simulink model "twolevel_seriesparallel"  (R2016a)
settings: Solver=VariableStepAuto  StartTime=0.0  StopTime=stop_time  RelTol=1e-3  AbsTol=1e-6
values from neighbouring files (symbols this model uses):
  DCLINK_Cap = 0.65*1.35*capacitorsabiti/sw_frequency    (= 0.000406115702479)    [loadvariation.m]    (also in trials.m = 1.35*capacitorsabiti/sw_frequency; twolevel_seriesparallel_analysis.m)
  Ef = Vln_rms*cos(Load_Angle)    [loadvariation.m]    (also in trials.m; twolevel_seriesparallel_analysis.m)
  intangle1 = 0    [loadvariation.m]    (also in trials.m; twolevel_seriesparallel_analysis.m)
  intangle2 = interleaving_angle    (= 180)    [loadvariation.m]    (also in trials.m = 360; twolevel_seriesparallel_analysis.m)
  intangle3 = 0    [loadvariation.m]    (also in trials.m; twolevel_seriesparallel_analysis.m)
  intangle4 = interleaving_angle    (= 180)    [loadvariation.m]    (also in trials.m = 360; twolevel_seriesparallel_analysis.m)
  Load_Angle = acos(Load_Power_Factor)    [loadvariation.m]    (also in trials.m; twolevel_seriesparallel_analysis.m)
  Ls = n*m*Xs/ref_frequency    [loadvariation.m]    (also in trials.m; twolevel_seriesparallel_analysis.m)
  ma = 0.9    [loadvariation.m]    (also in trials.m; twolevel_seriesparallel_analysis.m)
  ref_frequency = 2*pi*50    (= 314.159265359)    [loadvariation.m]    (also in trials.m; twolevel_seriesparallel_analysis.m)
  Sampling_time = 1/(100*sw_frequency)    (= 1.65289256198e-06)    [loadvariation.m]    (also in twolevel_seriesparallel_analysis.m = 8.26446280992e-06)
  Vin = DC_Voltage_Source + Rin*(Load_Real_Power/DC_Voltage_Source)    (= 554.814814815)    [loadvariation.m]    (also in trials.m; twolevel_seriesparallel_analysis.m)
undefined symbols (not defined in the file or in its folder): intangle5, intangle6, intangle7, intangle8, Lload, Rload
libraries: powerlib x106, powerlib_meascontrol x58, simulink x24
(part 2 of 2)

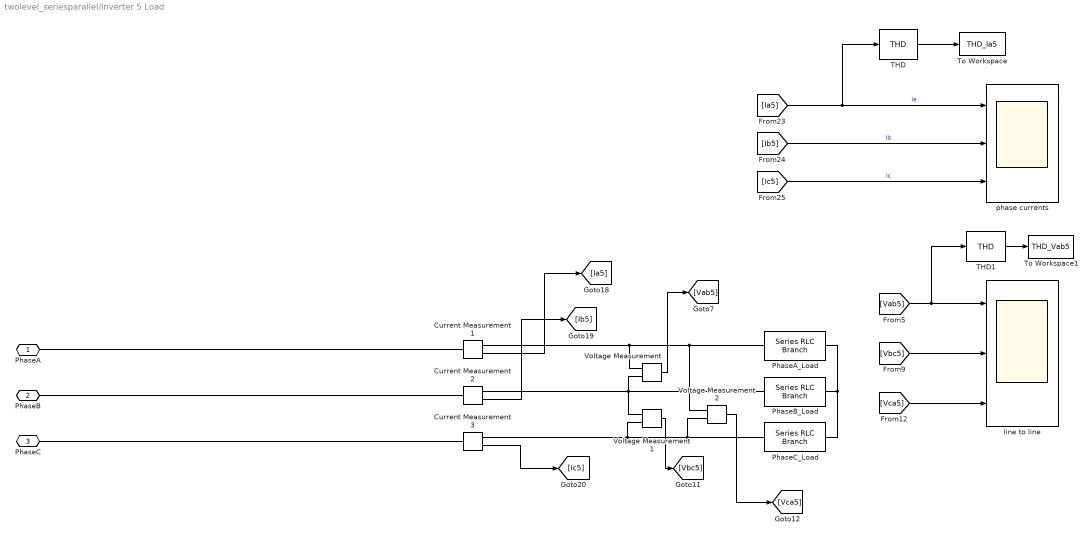
== system twolevel_seriesparallel/Inverter 5 Load ==
  Current Measurement1 : powerlib/Measurements/Current Measurement  PhasorSimulation=off  OutputType=Complex  PSBequivalent=0
  Current Measurement2 : powerlib/Measurements/Current Measurement  PhasorSimulation=off  OutputType=Complex  PSBequivalent=0
  Current Measurement3 : powerlib/Measurements/Current Measurement  PhasorSimulation=off  OutputType=Complex  PSBequivalent=0
  PhaseA_Load : powerlib/Elements/Series RLC Branch  LConnTagsString=__new0  RConnTagsString=__new0  BranchType=RL  Resistance=Rload  Inductance=Lload  SetiL0=off  InitialCurrent=0  Capacitance=1e-6  Setx0=off  InitialVoltage=0  Measurements=None
  PhaseB_Load : powerlib/Elements/Series RLC Branch  LConnTagsString=__new0  RConnTagsString=__new0  BranchType=RL  Resistance=Rload  Inductance=Lload  SetiL0=off  InitialCurrent=0  Capacitance=1e-6  Setx0=off  InitialVoltage=0  Measurements=None
  PhaseC_Load : powerlib/Elements/Series RLC Branch  LConnTagsString=__new0  RConnTagsString=__new0  BranchType=RL  Resistance=Rload  Inductance=Lload  SetiL0=off  InitialCurrent=0  Capacitance=1e-6  Setx0=off  InitialVoltage=0  Measurements=None
  THD : powerlib_meascontrol/Measurements/THD  Freq=Load_Nominal_Freq  Ts=0
  THD1 : powerlib_meascontrol/Measurements/THD  Freq=Load_Nominal_Freq  Ts=0
  To Workspace : ToWorkspace  VariableName=THD_Ia5  SaveFormat=Timeseries  SampleTime=-1
  To Workspace1 : ToWorkspace  VariableName=THD_Vab5  SaveFormat=Timeseries  SampleTime=-1
  Voltage Measurement : powerlib/Measurements/Voltage Measurement  PhasorSimulation=off  OutputType=Complex  PSBequivalent=0
  Voltage Measurement1 : powerlib/Measurements/Voltage Measurement  PhasorSimulation=off  OutputType=Complex  PSBequivalent=0
  Voltage Measurement2 : powerlib/Measurements/Voltage Measurement  PhasorSimulation=off  OutputType=Complex  PSBequivalent=0
  line to line : Scope  NumInputPorts=3
  phase currents : Scope  NumInputPorts=3
  PhaseA : PMIOPort  Port=1  Side=Left
  PhaseB : PMIOPort  Port=2  Side=Left
  PhaseC : PMIOPort  Port=3  Side=Left
  wires:
  THD1/1 -> To Workspace1/1
  [Ib5] -> phase currents/2  "Ib"
  Voltage Measurement2/1 -> [Vca5]
  THD/1 -> To Workspace/1
  [Vca5] -> line to line/3
  [Vab5] -> line to line/1, THD1/1
  [Vbc5] -> line to line/2
  [Ic5] -> phase currents/3  "Ic"
  [Ia5] -> phase currents/1, THD/1  "Ia"
  Current Measurement3/1 -> [Ic5]
  Voltage Measurement1/1 -> [Vbc5]
  Voltage Measurement/1 -> [Vab5]
  Current Measurement2/1 -> [Ib5]
  Current Measurement1/1 -> [Ia5]
  connections:
  PhaseA_Load/LConn1 -- Voltage Measurement2/LConn2 -- Voltage Measurement/LConn1 -- Current Measurement1/RConn1
  PhaseA/RConn1 -- Current Measurement1/LConn1
  Current Measurement2/LConn1 -- PhaseB/RConn1
  Current Measurement3/RConn1 -- Voltage Measurement1/LConn2 -- Voltage Measurement2/LConn1 -- PhaseC_Load/LConn1
  PhaseC/RConn1 -- Current Measurement3/LConn1
  PhaseC_Load/RConn1 -- PhaseB_Load/RConn1 -- PhaseA_Load/RConn1
  PhaseB_Load/LConn1 -- Voltage Measurement/LConn2 -- Voltage Measurement1/LConn1 -- Current Measurement2/RConn1

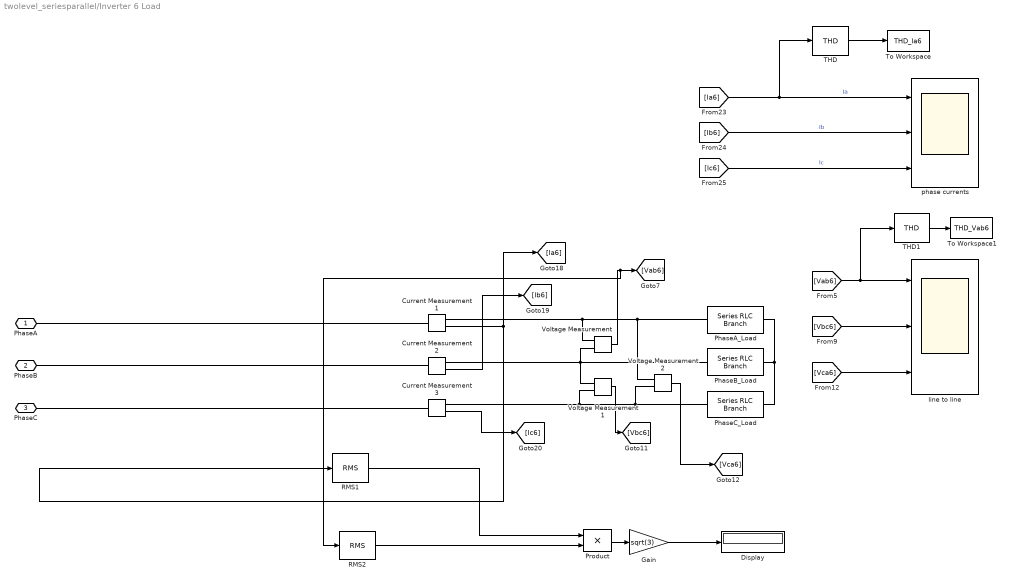
== system twolevel_seriesparallel/Inverter 6 Load ==
  Current Measurement1 : powerlib/Measurements/Current Measurement  PhasorSimulation=off  OutputType=Complex  PSBequivalent=0
  Current Measurement2 : powerlib/Measurements/Current Measurement  PhasorSimulation=off  OutputType=Complex  PSBequivalent=0
  Current Measurement3 : powerlib/Measurements/Current Measurement  PhasorSimulation=off  OutputType=Complex  PSBequivalent=0
  Display : Display
  Gain : Gain  Gain=sqrt(3)
  PhaseA_Load : powerlib/Elements/Series RLC Branch  LConnTagsString=__new0  RConnTagsString=__new0  BranchType=RL  Resistance=Rload  Inductance=Lload  SetiL0=off  InitialCurrent=0  Capacitance=1e-6  Setx0=off  InitialVoltage=0  Measurements=None
  PhaseB_Load : powerlib/Elements/Series RLC Branch  LConnTagsString=__new0  RConnTagsString=__new0  BranchType=RL  Resistance=Rload  Inductance=Lload  SetiL0=off  InitialCurrent=0  Capacitance=1e-6  Setx0=off  InitialVoltage=0  Measurements=None
  PhaseC_Load : powerlib/Elements/Series RLC Branch  LConnTagsString=__new0  RConnTagsString=__new0  BranchType=RL  Resistance=Rload  Inductance=Lload  SetiL0=off  InitialCurrent=0  Capacitance=1e-6  Setx0=off  InitialVoltage=0  Measurements=None
  Product : Product
  RMS1 : powerlib_meascontrol/Measurements/RMS  TrueRMS=on  Freq=Load_Nominal_Freq  RMSInit=120  Ts=0
  RMS2 : powerlib_meascontrol/Measurements/RMS  TrueRMS=on  Freq=Load_Nominal_Freq  RMSInit=120  Ts=0
  THD : powerlib_meascontrol/Measurements/THD  Freq=Load_Nominal_Freq  Ts=0
  THD1 : powerlib_meascontrol/Measurements/THD  Freq=Load_Nominal_Freq  Ts=0
  To Workspace : ToWorkspace  VariableName=THD_Ia6  SaveFormat=Timeseries  SampleTime=-1
  To Workspace1 : ToWorkspace  VariableName=THD_Vab6  SaveFormat=Timeseries  SampleTime=-1
  Voltage Measurement : powerlib/Measurements/Voltage Measurement  PhasorSimulation=off  OutputType=Complex  PSBequivalent=0
  Voltage Measurement1 : powerlib/Measurements/Voltage Measurement  PhasorSimulation=off  OutputType=Complex  PSBequivalent=0
  Voltage Measurement2 : powerlib/Measurements/Voltage Measurement  PhasorSimulation=off  OutputType=Complex  PSBequivalent=0
  line to line : Scope  NumInputPorts=3
  phase currents : Scope  NumInputPorts=3
  PhaseA : PMIOPort  Port=1  Side=Left
  PhaseB : PMIOPort  Port=2  Side=Left
  PhaseC : PMIOPort  Port=3  Side=Left
  wires:
  Current Measurement1/1 -> [Ia6], RMS1/1
  Current Measurement2/1 -> [Ib6]
  Voltage Measurement/1 -> RMS2/1, [Vab6]
  Voltage Measurement1/1 -> [Vbc6]
  Current Measurement3/1 -> [Ic6]
  [Ia6] -> THD/1, phase currents/1  "Ia"
  [Ic6] -> phase currents/3  "Ic"
  [Vbc6] -> line to line/2
  [Vab6] -> THD1/1, line to line/1
  [Vca6] -> line to line/3
  THD/1 -> To Workspace/1
  Voltage Measurement2/1 -> [Vca6]
  [Ib6] -> phase currents/2  "Ib"
  THD1/1 -> To Workspace1/1
  Product/1 -> Gain/1
  RMS1/1 -> Product/1
  RMS2/1 -> Product/2
  Gain/1 -> Display/1
  connections:
  Current Measurement2/RConn1 -- Voltage Measurement1/LConn1 -- Voltage Measurement/LConn2 -- PhaseB_Load/LConn1
  PhaseA_Load/RConn1 -- PhaseB_Load/RConn1 -- PhaseC_Load/RConn1
  PhaseC/RConn1 -- Current Measurement3/LConn1
  PhaseC_Load/LConn1 -- Voltage Measurement2/LConn1 -- Voltage Measurement1/LConn2 -- Current Measurement3/RConn1
  Current Measurement2/LConn1 -- PhaseB/RConn1
  PhaseA/RConn1 -- Current Measurement1/LConn1
  Current Measurement1/RConn1 -- Voltage Measurement/LConn1 -- Voltage Measurement2/LConn2 -- PhaseA_Load/LConn1

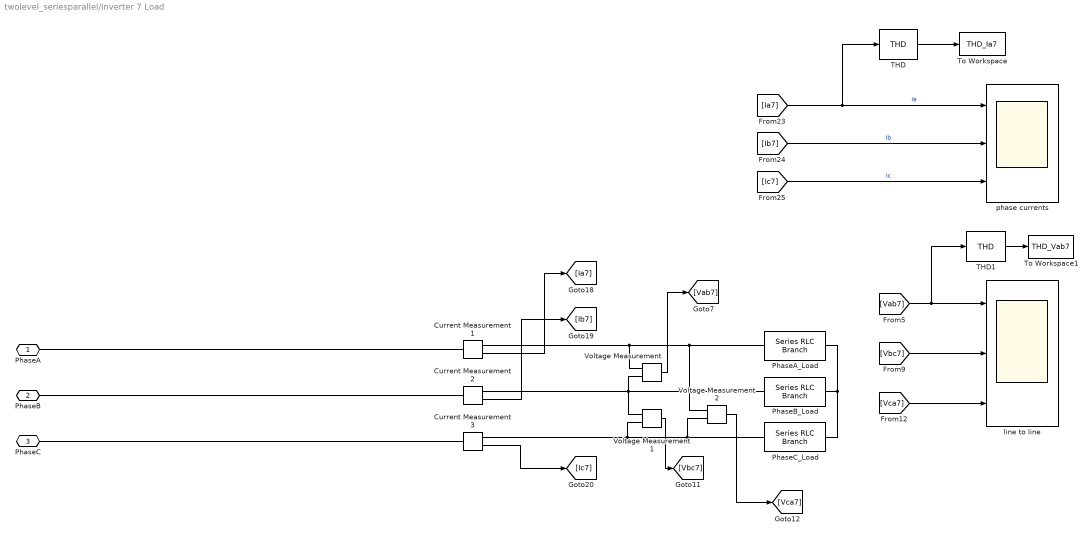
== system twolevel_seriesparallel/Inverter 7 Load ==
  Current Measurement1 : powerlib/Measurements/Current Measurement  PhasorSimulation=off  OutputType=Complex  PSBequivalent=0
  Current Measurement2 : powerlib/Measurements/Current Measurement  PhasorSimulation=off  OutputType=Complex  PSBequivalent=0
  Current Measurement3 : powerlib/Measurements/Current Measurement  PhasorSimulation=off  OutputType=Complex  PSBequivalent=0
  PhaseA_Load : powerlib/Elements/Series RLC Branch  LConnTagsString=__new0  RConnTagsString=__new0  BranchType=RL  Resistance=Rload  Inductance=Lload  SetiL0=off  InitialCurrent=0  Capacitance=1e-6  Setx0=off  InitialVoltage=0  Measurements=None
  PhaseB_Load : powerlib/Elements/Series RLC Branch  LConnTagsString=__new0  RConnTagsString=__new0  BranchType=RL  Resistance=Rload  Inductance=Lload  SetiL0=off  InitialCurrent=0  Capacitance=1e-6  Setx0=off  InitialVoltage=0  Measurements=None
  PhaseC_Load : powerlib/Elements/Series RLC Branch  LConnTagsString=__new0  RConnTagsString=__new0  BranchType=RL  Resistance=Rload  Inductance=Lload  SetiL0=off  InitialCurrent=0  Capacitance=1e-6  Setx0=off  InitialVoltage=0  Measurements=None
  THD : powerlib_meascontrol/Measurements/THD  Freq=Load_Nominal_Freq  Ts=0
  THD1 : powerlib_meascontrol/Measurements/THD  Freq=Load_Nominal_Freq  Ts=0
  To Workspace : ToWorkspace  VariableName=THD_Ia7  SaveFormat=Timeseries  SampleTime=-1
  To Workspace1 : ToWorkspace  VariableName=THD_Vab7  SaveFormat=Timeseries  SampleTime=-1
  Voltage Measurement : powerlib/Measurements/Voltage Measurement  PhasorSimulation=off  OutputType=Complex  PSBequivalent=0
  Voltage Measurement1 : powerlib/Measurements/Voltage Measurement  PhasorSimulation=off  OutputType=Complex  PSBequivalent=0
  Voltage Measurement2 : powerlib/Measurements/Voltage Measurement  PhasorSimulation=off  OutputType=Complex  PSBequivalent=0
  line to line : Scope  NumInputPorts=3
  phase currents : Scope  NumInputPorts=3
  PhaseA : PMIOPort  Port=1  Side=Left
  PhaseB : PMIOPort  Port=2  Side=Left
  PhaseC : PMIOPort  Port=3  Side=Left
  wires:
  Current Measurement1/1 -> [Ia7]
  Current Measurement2/1 -> [Ib7]
  Voltage Measurement/1 -> [Vab7]
  Voltage Measurement1/1 -> [Vbc7]
  Current Measurement3/1 -> [Ic7]
  [Ia7] -> THD/1, phase currents/1  "Ia"
  [Ic7] -> phase currents/3  "Ic"
  [Vbc7] -> line to line/2
  [Vab7] -> THD1/1, line to line/1
  [Vca7] -> line to line/3
  THD/1 -> To Workspace/1
  Voltage Measurement2/1 -> [Vca7]
  [Ib7] -> phase currents/2  "Ib"
  THD1/1 -> To Workspace1/1
  connections:
  Current Measurement2/RConn1 -- Voltage Measurement1/LConn1 -- Voltage Measurement/LConn2 -- PhaseB_Load/LConn1
  PhaseA_Load/RConn1 -- PhaseB_Load/RConn1 -- PhaseC_Load/RConn1
  PhaseC/RConn1 -- Current Measurement3/LConn1
  PhaseC_Load/LConn1 -- Voltage Measurement2/LConn1 -- Voltage Measurement1/LConn2 -- Current Measurement3/RConn1
  Current Measurement2/LConn1 -- PhaseB/RConn1
  PhaseA/RConn1 -- Current Measurement1/LConn1
  Current Measurement1/RConn1 -- Voltage Measurement/LConn1 -- Voltage Measurement2/LConn2 -- PhaseA_Load/LConn1

== system twolevel_seriesparallel/Inverter 8 Load ==
  Current Measurement1 : powerlib/Measurements/Current Measurement  PhasorSimulation=off  OutputType=Complex  PSBequivalent=0
  Current Measurement2 : powerlib/Measurements/Current Measurement  PhasorSimulation=off  OutputType=Complex  PSBequivalent=0
  Current Measurement3 : powerlib/Measurements/Current Measurement  PhasorSimulation=off  OutputType=Complex  PSBequivalent=0
  PhaseA_Load : powerlib/Elements/Series RLC Branch  LConnTagsString=__new0  RConnTagsString=__new0  BranchType=RL  Resistance=Rload  Inductance=Lload  SetiL0=off  InitialCurrent=0  Capacitance=1e-6  Setx0=off  InitialVoltage=0  Measurements=None
  PhaseB_Load : powerlib/Elements/Series RLC Branch  LConnTagsString=__new0  RConnTagsString=__new0  BranchType=RL  Resistance=Rload  Inductance=Lload  SetiL0=off  InitialCurrent=0  Capacitance=1e-6  Setx0=off  InitialVoltage=0  Measurements=None
  PhaseC_Load : powerlib/Elements/Series RLC Branch  LConnTagsString=__new0  RConnTagsString=__new0  BranchType=RL  Resistance=Rload  Inductance=Lload  SetiL0=off  InitialCurrent=0  Capacitance=1e-6  Setx0=off  InitialVoltage=0  Measurements=None
  THD : powerlib_meascontrol/Measurements/THD  Freq=Load_Nominal_Freq  Ts=0
  THD1 : powerlib_meascontrol/Measurements/THD  Freq=Load_Nominal_Freq  Ts=0
  To Workspace : ToWorkspace  VariableName=THD_Ia8  SaveFormat=Timeseries  SampleTime=-1
  To Workspace1 : ToWorkspace  VariableName=THD_Vab8  SaveFormat=Timeseries  SampleTime=-1
  Voltage Measurement : powerlib/Measurements/Voltage Measurement  PhasorSimulation=off  OutputType=Complex  PSBequivalent=0
  Voltage Measurement1 : powerlib/Measurements/Voltage Measurement  PhasorSimulation=off  OutputType=Complex  PSBequivalent=0
  Voltage Measurement2 : powerlib/Measurements/Voltage Measurement  PhasorSimulation=off  OutputType=Complex  PSBequivalent=0
  line to line : Scope  NumInputPorts=3
  phase currents : Scope  NumInputPorts=3
  PhaseA : PMIOPort  Port=1  Side=Left
  PhaseB : PMIOPort  Port=2  Side=Left
  PhaseC : PMIOPort  Port=3  Side=Left
  wires:
  THD1/1 -> To Workspace1/1
  [Ib8] -> phase currents/2  "Ib"
  Voltage Measurement2/1 -> [Vca8]
  THD/1 -> To Workspace/1
  [Vca8] -> line to line/3
  [Vab8] -> line to line/1, THD1/1
  [Vbc8] -> line to line/2
  [Ic8] -> phase currents/3  "Ic"
  [Ia8] -> phase currents/1, THD/1  "Ia"
  Current Measurement3/1 -> [Ic8]
  Voltage Measurement1/1 -> [Vbc8]
  Voltage Measurement/1 -> [Vab8]
  Current Measurement2/1 -> [Ib8]
  Current Measurement1/1 -> [Ia8]
  connections:
  PhaseA_Load/LConn1 -- Voltage Measurement2/LConn2 -- Voltage Measurement/LConn1 -- Current Measurement1/RConn1
  PhaseA/RConn1 -- Current Measurement1/LConn1
  Current Measurement2/LConn1 -- PhaseB/RConn1
  Current Measurement3/RConn1 -- Voltage Measurement1/LConn2 -- Voltage Measurement2/LConn1 -- PhaseC_Load/LConn1
  PhaseC/RConn1 -- Current Measurement3/LConn1
  PhaseC_Load/RConn1 -- PhaseB_Load/RConn1 -- PhaseA_Load/RConn1
  PhaseB_Load/LConn1 -- Voltage Measurement/LConn2 -- Voltage Measurement1/LConn1 -- Current Measurement2/RConn1
